simulink model "Makerspace_Schematic"  (R2021a)
settings: Solver=VariableStepAuto  StartTime=0.0  StopTime=10.0  RelTol=1e-3
settings Model: Creator=sandhyanatarajan  LastModifiedBy=sandhyanatarajan

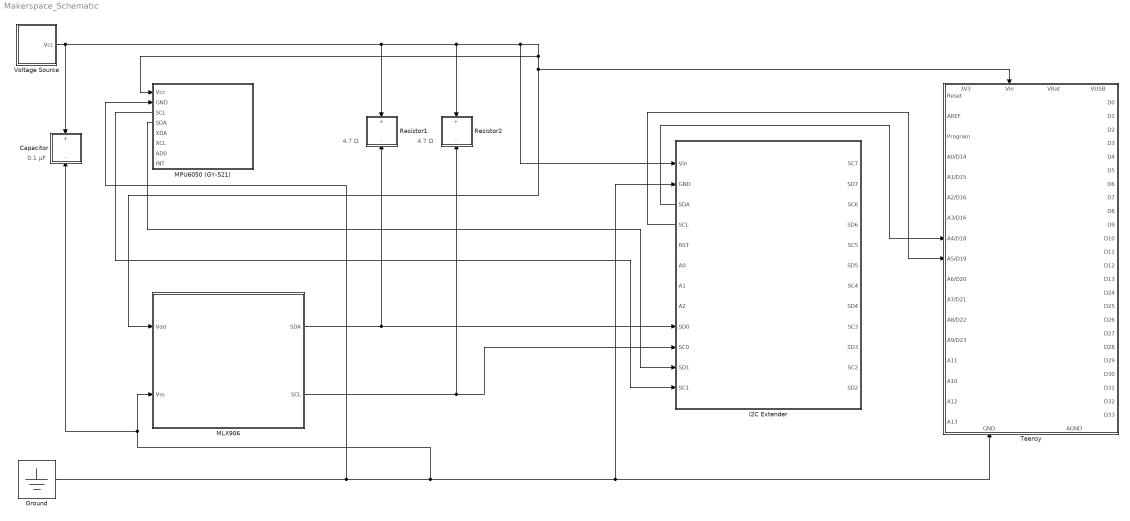
== system Makerspace_Schematic ==
  note: 0.1 µF
  note: 4.7 Ω
  note: 4.7 Ω
  Capacitor : Subsystem
      settings: PortSchema="{\"entries\":[{\"content\":{\"sides\":[{\"content\":{\"connectorIds\":[\"In1\"]},\"type\":\"ConnectorPlacement.EquallySpacedRectSide\",\"uuid\":\"599f6337-b0b4-455f-abe6-702e754742c2\"},{\"content\":{\"connectorIds\":[\"In2\"],\"side\":\"RIGHT\"},\"type\":\"ConnectorPlacement.EquallySpacedRectSide\",\"uuid\":\"64ca4af4-916e-47c5-ad53-6c8fdaaada72\"},{\"content\":{\"connectorIds\":[],\"side\":\"TOP\"},\"type\":\"ConnectorPlacement.EquallySpacedRectSide\",\"uuid\":\"a77af66a-ffb7-407d-8dbc-9ba25ed7f745\"}]},\"type\":\"ConnectorPlacement.EquallySpacedConnector\",\"uuid\":\"dd4d65e5-3bef-4431-be96-be4c9d8ec1db\"}],\"packageUris\":[\"http://schema.mathworks.com/mf0/Connector/R2020b\"],\"version\":\"1.0\"}"
  Ground : Ground
  I2C Extender : Subsystem
      settings: PortSchema="{\"entries\":[{\"content\":{\"sides\":[{\"content\":{\"connectorIds\":[\"In1\",\"In2\",\"Out1\",\"Out2\",\"In3\",\"In4\",\"In5\",\"In6\",\"In7\",\"In8\",\"In9\",\"In10\"]},\"type\":\"ConnectorPlacement.EquallySpacedRectSide\",\"uuid\":\"a6c6577c-3c13-4581-9c08-1cf3147c0a5b\"},{\"content\":{\"connectorIds\":[\"In11\",\"In12\",\"In13\",\"In14\",\"In15\",\"In16\",\"In17\",\"In18\",\"In19\",\"In20\",\"In21\",\"In22\"],\"side\":\"RIGHT\"},\"type\":\"ConnectorPlacement.EquallySpacedRectSide\",\"uuid\":\"2fb759a8-b7f0-42f0-8c86-8b18b4156499\"},{\"content\":{\"connectorIds\":[],\"side\":\"TOP\"},\"type\":\"ConnectorPlacement.EquallySpacedRectSide\",\"uuid\":\"65b217a8-f894-4818-961b-3514861ada67\"}]},\"type\":\"ConnectorPlacement.EquallySpacedConnector\",\"uuid\":\"db0ed37c-26ef-4a78-98d4-8cb94eb84801\"}],\"packageUris\":[\"http://schema.mathworks.com/mf0/Connector/R2020b\"],\"version\":\"1.0\"}"
  MLX906 : Subsystem
  MPU6050 (GY-521) : Subsystem
      settings: PortSchema="{\"entries\":[{\"content\":{\"sides\":[{\"content\":{\"connectorIds\":[\"In1\",\"In2\",\"Out1\",\"Out2\",\"Out3\",\"Out4\",\"Out5\",\"Out6\"]},\"type\":\"ConnectorPlacement.EquallySpacedRectSide\",\"uuid\":\"6e0e29fc-5c98-4283-9c5e-63e6a78d3862\"},{\"content\":{\"connectorIds\":[],\"side\":\"RIGHT\"},\"type\":\"ConnectorPlacement.EquallySpacedRectSide\",\"uuid\":\"ea4a38e6-80fe-4eb3-af66-ed78145396de\"},{\"content\":{\"connectorIds\":[],\"side\":\"TOP\"},\"type\":\"ConnectorPlacement.EquallySpacedRectSide\",\"uuid\":\"55af817d-f73b-4403-b785-13330552a87f\"}]},\"type\":\"ConnectorPlacement.EquallySpacedConnector\",\"uuid\":\"c3c138ff-f01e-433a-953d-d370cb614218\"}],\"packageUris\":[\"http://schema.mathworks.com/mf0/Connector/R2020b\"],\"version\":\"1.0\"}"
  Resistor1 : Subsystem
      settings: PortSchema="{\"entries\":[{\"content\":{\"sides\":[{\"content\":{\"connectorIds\":[\"In1\"]},\"type\":\"ConnectorPlacement.EquallySpacedRectSide\",\"uuid\":\"599f6337-b0b4-455f-abe6-702e754742c2\"},{\"content\":{\"connectorIds\":[\"In2\"],\"side\":\"RIGHT\"},\"type\":\"ConnectorPlacement.EquallySpacedRectSide\",\"uuid\":\"64ca4af4-916e-47c5-ad53-6c8fdaaada72\"},{\"content\":{\"connectorIds\":[],\"side\":\"TOP\"},\"type\":\"ConnectorPlacement.EquallySpacedRectSide\",\"uuid\":\"a77af66a-ffb7-407d-8dbc-9ba25ed7f745\"}]},\"type\":\"ConnectorPlacement.EquallySpacedConnector\",\"uuid\":\"dd4d65e5-3bef-4431-be96-be4c9d8ec1db\"}],\"packageUris\":[\"http://schema.mathworks.com/mf0/Connector/R2020b\"],\"version\":\"1.0\"}"
  Resistor2 : Subsystem
      settings: PortSchema="{\"entries\":[{\"content\":{\"sides\":[{\"content\":{\"connectorIds\":[\"In1\"]},\"type\":\"ConnectorPlacement.EquallySpacedRectSide\",\"uuid\":\"599f6337-b0b4-455f-abe6-702e754742c2\"},{\"content\":{\"connectorIds\":[\"In2\"],\"side\":\"RIGHT\"},\"type\":\"ConnectorPlacement.EquallySpacedRectSide\",\"uuid\":\"64ca4af4-916e-47c5-ad53-6c8fdaaada72\"},{\"content\":{\"connectorIds\":[],\"side\":\"TOP\"},\"type\":\"ConnectorPlacement.EquallySpacedRectSide\",\"uuid\":\"a77af66a-ffb7-407d-8dbc-9ba25ed7f745\"}]},\"type\":\"ConnectorPlacement.EquallySpacedConnector\",\"uuid\":\"dd4d65e5-3bef-4431-be96-be4c9d8ec1db\"}],\"packageUris\":[\"http://schema.mathworks.com/mf0/Connector/R2020b\"],\"version\":\"1.0\"}"
  Teensy : Subsystem
      settings: PortSchema="{\"entries\":[{\"content\":{\"sides\":[{\"content\":{\"connectorIds\":[\"In1\",\"In2\",\"In3\",\"In4\",\"In5\",\"In6\",\"In7\",\"In8\",\"In9\",\"In10\",\"In11\",\"In12\",\"In13\",\"In14\",\"In15\",\"In16\",\"In17\"]},\"type\":\"ConnectorPlacement.EquallySpacedRectSide\",\"uuid\":\"73aca493-1339-456c-a89c-762982cb69f1\"},{\"content\":{\"connectorIds\":[\"Out1\",\"Out2\",\"Out3\",\"Out4\",\"Out5\",\"Out6\",\"Out7\",\"Out8\",\"Out9\",\"Out10\",\"Out11\",\"Out12\",\"Out13\",\"Out14\",\"Out15\",\"Out16\",\"Out17\",\"Out18\",\"Out19\",\"Out20\",\"Out21\",\"Out22\",\"Out23\",\"Out24\"],\"side\":\"RIGHT\"},\"type\":\"ConnectorPlacement.EquallySpacedRectSide\",\"uuid\":\"62bb247c-1d8d-4a4d-bce9-e073d97c55f3\"},{\"content\":{\"connectorIds\":[\"In18\",\"In19\",\"In20\",\"In21\"],\"side\":\"TOP\"},\"type\":\"ConnectorPlacement.EquallySpacedRectSide\",\"uuid\":\"9db3a753-1af2-4118-b74f-31e133181e86\"},{\"content\":{\"connectorIds\":[\"In22\",\"In23\"],\"side\":\"BOTTOM\"},\"type\":\"ConnectorPlacement.EquallySpacedRectSide\",\"uuid\":\"90a64c3c-a3e0-4cd4-bb40-849f306030f0\"}]},\"type\":\"ConnectorPlacement.EquallySpacedConnector\",\"uuid\":\"bf657516-4018-4e75-ba14-3e57b59466f7\"}],\"packageUris\":[\"http://schema.mathworks.com/mf0/Connector/R2020b\"],\"version\":\"1.0\"}"
  Voltage Source : Subsystem
  wires:
  Ground/1 -> Teensy/22(GND), I2C Extender/2(GND), Capacitor/2(-), MLX906/2(Vss), MPU6050 (GY-521)/2(GND)
  I2C Extender/1(SDA) -> Teensy/8(A4/D18)
  I2C Extender/2(SCL) -> Teensy/9(A5/D19)
  MLX906/1(SDA) -> I2C Extender/7(SD0), Resistor1/2(-)
  MLX906/2(SCL) -> Resistor2/2(-), I2C Extender/8(SC0)
  MPU6050 (GY-521)/1(SCL) -> I2C Extender/10(SC1)
  MPU6050 (GY-521)/2(SDA) -> I2C Extender/9(SD1)
  Voltage Source/1(Vcc) -> Resistor2/1(+), Teensy/19(Vin), MLX906/1(Vdd), MPU6050 (GY-521)/1(Vcc), I2C Extender/1(Vin), Resistor1/1(+), Capacitor/1(+)

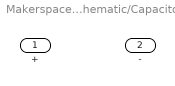
== system Makerspace_Schematic/Capacitor ==
  + : Inport
  - : Inport  Port=2

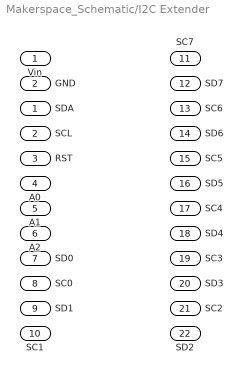
== system Makerspace_Schematic/I2C Extender ==
  Vin : Inport
  GND : Inport  Port=2
  RST : Inport  Port=3
  A0 : Inport  Port=4
  A1 : Inport  Port=5
  A2 : Inport  Port=6
  SD0 : Inport  Port=7
  SC0 : Inport  Port=8
  SD1 : Inport  Port=9
  SC1 : Inport  Port=10
  SC7 : Inport  Port=11
  SD7 : Inport  Port=12
  SC6 : Inport  Port=13
  SD6 : Inport  Port=14
  SC5 : Inport  Port=15
  SD5 : Inport  Port=16
  SC4 : Inport  Port=17
  SD4 : Inport  Port=18
  SC3 : Inport  Port=19
  SD3 : Inport  Port=20
  SC2 : Inport  Port=21
  SD2 : Inport  Port=22
  SDA : Outport
  SCL : Outport  Port=2

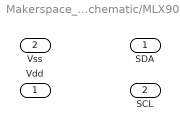
== system Makerspace_Schematic/MLX906 ==
  Vdd : Inport
  Vss : Inport  Port=2
  SDA : Outport
  SCL : Outport  Port=2

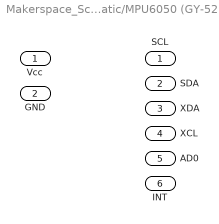
== system Makerspace_Schematic/MPU6050 (GY-521) ==
  Vcc : Inport
  GND : Inport  Port=2
  SCL : Outport
  SDA : Outport  Port=2
  XDA : Outport  Port=3
  XCL : Outport  Port=4
  AD0 : Outport  Port=5
  INT : Outport  Port=6

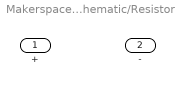
== system Makerspace_Schematic/Resistor1 ==
  + : Inport
  - : Inport  Port=2

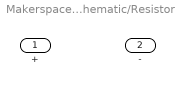
== system Makerspace_Schematic/Resistor2 ==
  + : Inport
  - : Inport  Port=2

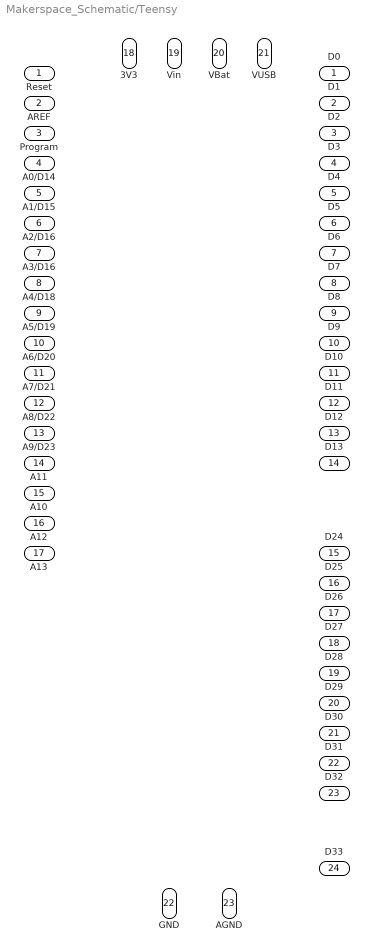
== system Makerspace_Schematic/Teensy ==
  Reset : Inport
  AREF : Inport  Port=2
  Program : Inport  Port=3
  A0/D14 : Inport  Port=4
  A1/D15 : Inport  Port=5
  A2/D16 : Inport  Port=6
  A3/D16 : Inport  Port=7
  A4/D18 : Inport  Port=8
  A5/D19 : Inport  Port=9
  A6/D20 : Inport  Port=10
  A7/D21 : Inport  Port=11
  A8/D22 : Inport  Port=12
  A9/D23 : Inport  Port=13
  A11 : Inport  Port=14
  A10 : Inport  Port=15
  A12 : Inport  Port=16
  A13 : Inport  Port=17
  3V3 : Inport  Port=18
  Vin : Inport  Port=19
  VBat : Inport  Port=20
  VUSB : Inport  Port=21
  GND : Inport  Port=22
  AGND : Inport  Port=23
  D0 : Outport
  D1 : Outport  Port=2
  D2 : Outport  Port=3
  D3 : Outport  Port=4
  D4 : Outport  Port=5
  D5 : Outport  Port=6
  D6 : Outport  Port=7
  D7 : Outport  Port=8
  D8 : Outport  Port=9
  D9 : Outport  Port=10
  D10 : Outport  Port=11
  D11 : Outport  Port=12
  D12 : Outport  Port=13
  D13 : Outport  Port=14
  D24 : Outport  Port=15
  D25 : Outport  Port=16
  D26 : Outport  Port=17
  D27 : Outport  Port=18
  D28 : Outport  Port=19
  D29 : Outport  Port=20
  D30 : Outport  Port=21
  D31 : Outport  Port=22
  D32 : Outport  Port=23
  D33 : Outport  Port=24

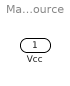
== system Makerspace_Schematic/Voltage Source ==
  Vcc : Outport
